simulink model "part_depth2"  (R2023a)
settings: Solver=VariableStepAuto  StartTime=0.0  StopTime=10.0  RelTol=1e-3
libraries: dspvision x1, visiongeotforms x1, visionsinks x1
settings Model: Creator=Asus  LastModifiedBy=Asus
settings SFSimCC: SimTargetLang=C++

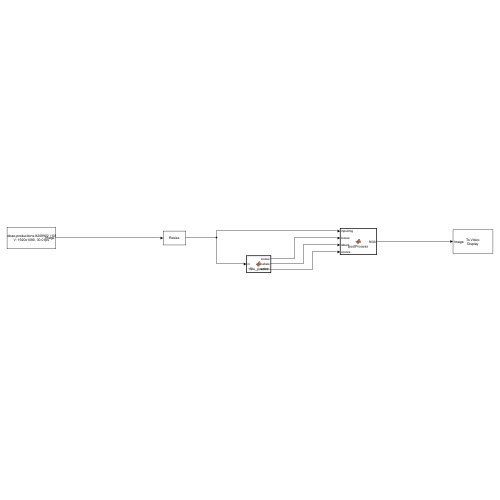
[thumbnail: Simulink's stored preview of the top-level diagram]
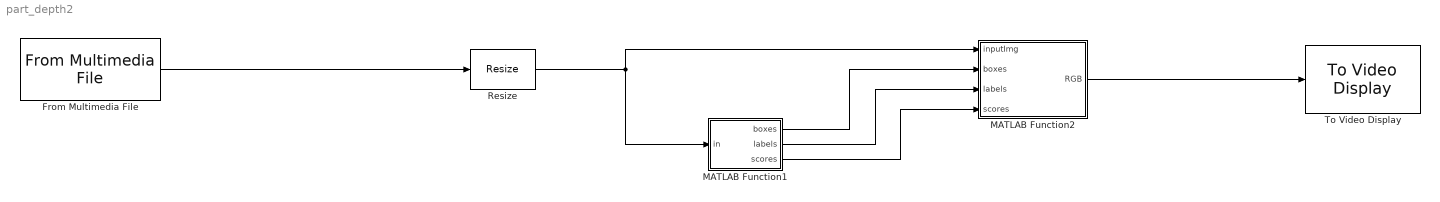
== system part_depth2 ==
  From Multimedia File : dspvision/From Multimedia File  inputFilename=C:\Users\Asus\MATLAB Drive\RVP_SIR_INTERN_PROJECT\pexels-rodnae-productions-8208902 (1080p).mp4  readRange=[1 Inf]  loop=on  numPlays=inf  outputStreams=Video only  videoDataType=uint8  audioDataType=int16  inheritSampleTime=on  userDefinedSampleTime=1/30  noAudioOutput=off  isIntensityVideo=off  fourcc=RGB  colorVideoFormat=One multidimensional signal  outputEOF=off  dataOrg=Column-major  audioFrameSize=1024  computeAudioFrameSize=off  outSamplingMode=Sample based
      settings: LibrarySourceBlock=visionsources/From Multimedia File
  MATLAB Function1 : MATLAB Function  TreatAsAtomicUnit=on
  MATLAB Function2 : MATLAB Function  TreatAsAtomicUnit=on
  Resize : visiongeotforms/Resize  specify=Number of output rows and columns  rfactor=[200 150]  outCols=25  outRows=25  outRowsCols=[256 256]  interp_method=Bilinear  antialias=on  useROI=off  roiFlag=off  roundingMode=Nearest  overflowMode=on  prodOutputMode=Binary point scaling  prodOutputWordLength=32  prodOutputFracLength=10
  To Video Display : visionsinks/To Video Display  windowSizeMode=Normal  openAtMdlStart=on  fullScreen=off  videoWindowX=536805376  videoWindowY=536805376  saveWindowSize=off  videoWindowWidth=2147483647  videoWindowHeight=2147483647  inputColorFormat=RGB  inputType=Obsolete  imagePorts=One multidimensional signal  OutputDevice=On-screen video monitor  dataOrg=Column-major  isWindowOpen=off
  wires:
  MATLAB Function2/1(RGB) -> To Video Display/1
  MATLAB Function1/2(labels) -> MATLAB Function2/3(labels)
  Resize/1 -> MATLAB Function2/1(inputImg), MATLAB Function1/1(in)
  MATLAB Function1/3(scores) -> MATLAB Function2/4(scores)
  MATLAB Function1/1(boxes) -> MATLAB Function2/2(boxes)
  From Multimedia File/1 -> Resize/1

== matlab function part_depth2/MATLAB Function1 ==
  data: in input; boxes output; labels output; scores output
function [boxes,labels,scores] = tflite_predict(in)
persistent net;
if isempty(net)
    net = loadTFLiteModel('lite-model_qat_mobilenet_v2_retinanet_256_1.tflite');
end
 net.NumThreads=4;
[boxes, labels, scores, ~] = predict(net, in, 'EnableINT8InferenceOnWindows', true);

== matlab function part_depth2/MATLAB Function2 ==
  data: inputImg input; RGB output; boxes input; labels input; scores input
function RGB = postProcess(inputImg, boxes, labels, scores)
    labelsFile = cell(80, 1); % Remove unnecessary cell initialization
    fid = fopen('label.txt');
    lne = myfgetl(fid);
    for i = 1:80
        labelsFile{i} = lne;
        lne = myfgetl(fid);
    end
    fclose(fid);
    labelsFile = readtxtFile(labelsFile);

    ymin = boxes(:, 1) * size(inputImg, 1);
    xmin = boxes(:, 2) * size(inputImg, 2);
    ymax = boxes(:, 3) * size(inputImg, 1);
    xmax = boxes(:, 4) * size(inputImg, 2);
    
    width = xmax - xmin;
    height = ymax - ymin;
    
     %%numBoxes = size(scores, 1);
    position = zeros(size(scores, 1), 4, 'single');
    labelVector = zeros(1, size(scores, 1), 'single');
    for i = 1:size(scores, 1)  % Use size(scores, 1) instead of numel(scores)
        position(i, 1:4) = [xmin(i), ymin(i), width(i), height(i)];
        labelVector(i) = labels(i) + 2; % Use i instead of 1 as the index
    end
    
    %numSelected = min(4, numBoxes);
    [selectedBbox, selectedScore, ~] = selectStrongestBbox(position, scores, 'NumStrongest', 4);
    
    labelCell = cell(4, 1);
    labelsArray = cell(4, 1);
    for i = 1:numel(labelCell)
        labelCell{i} = labelsFile{labelVector(i)};
        labelsArray{i} = [char(labelCell{i}), ':', char(sprintf('%.3g', selectedScore(i) * 100)), '%'];
    end
    
    RGB = insertObjectAnnotation(im2uint8(inputImg), 'rectangle', selectedBbox, labelsArray, 'FontSize', 13);
end

function [labelArray,lne] = readtxtFile(labelArray)
    fid = fopen('label.txt');
    lne = myfgetl(fid);
    count = 1;
% while ~isempty(lne)
     for i = 1:80
         labelArray{count} = lne;
         lne = myfgetl(fid);
         count = count + 1;
     end
     fclose(fid);
end

function line = myfgetl(fid)
    line = '';
    c = fread(fid, 1, 'char=>char');
    while ~feof(fid) && ~strcmp(c, newline)
        if ~strcmp(c, sprintf('\r'))
            line = [line, c];
        end
        c = fread(fid, 1, 'char=>char');
    end
end
